simulink model "test_sys"  (R2022a)
settings: Solver=FixedStepDiscrete  StartTime=0.0  StopTime=T_final  FixedStep=T_sample  RelTol=1e-3
values from neighbouring files (symbols this model uses):
  A = [0.921 0 0.041 0 ... (first row only)    [test.m]
  B = [0.017 0.001 ... (first row only)    [test.m]
  C = [1 0 0 0 ... (first row only)    [test.m]
  D = zeros(n_meas,n_int)    [test.m]
  x0 = [7;7]    [Run_model.m]    (also in prepare_trajectory_data.m; test.m = rand(n_states,1))
settings Model: Creator=Abelb  LastModifiedBy=Abely
settings DebuggingCC: UnconnectedInputMsg=warning  UnconnectedOutputMsg=warning  UnconnectedLineMsg=warning
settings RTWCC: DLArmComputeVersion=19.05

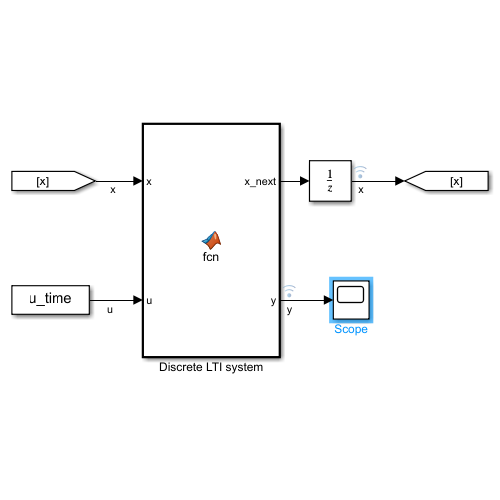
[thumbnail: Simulink's stored preview of the top-level diagram]
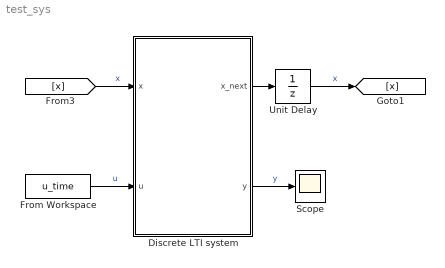
== system test_sys ==
  Discrete LTI system : MATLAB Function  TreatAsAtomicUnit=on
  From Workspace : FromWorkspace  VariableName=u_time
  Scope : Scope
  Unit Delay : UnitDelay  InitialCondition=x0  SampleTime=-1  HasFrameUpgradeWarning=on
  wires:
  Discrete LTI system/1(x_next) -> Unit Delay/1
  From Workspace/1 -> Discrete LTI system/2(u)  "u"
  Unit Delay/1 -> [x]  "x"
  [x] -> Discrete LTI system/1(x)  "x"
  Discrete LTI system/2(y) -> Scope/1  "y"

== matlab function test_sys/Discrete LTI system ==
  data: x input; x_next output; u input; y output; A parameter; C parameter; B parameter; D parameter
function [x_next,y] = fcn(x,u,A,C,B,D)
% Discrete state-space model for system

x_next = A*x + B*u;

y = C*x + D*u;
